simulink model "Multiplicative_Kalman_FullSystem"  (R2024a)
settings: Solver=FixedStepAuto  StartTime=0.0  StopTime=0.05  FixedStep=0.05  RelTol=1e-3
model workspace (MAT data in the model file):
  Delta_t = 0.1
  J1 = 0.1
  J2 = 0.13
  J3 = 0.05
  NoiseCov = [0.5  0  0  0  0  0; 0  0.5  0  0  0  0; 0  0  0.5  0  0  0; 0  0  0  0.5  0  0; 0  0  0  0  0.5  0; 0  0  0  0  0  0.5]
  Orbit_Incl = 51.6
  Q_identity = [0.05  0  0  0  0  0  0; 0  0.05  0  0  0  0  0; 0  0  0.05  0  0  0  0; 0  0  0  0.05  0  0  0; 0  0  0  0  0.05  0  0; 0  0  0  0  0  0.05  0; 0  0  0  0  0  0  0.05]
  Sig = Simulink.Signal
  Sig.DataType = 'auto'
  Sig.Dimensions = -1
  Sig.DimensionsMode = 'auto'
  Sig.Complexity = 'auto'
  Sig.SampleTime = -1
  Sig.SamplingMode = 'auto'
  controlRun = 1
  jd_input = 2458850
  m = 12
  n = 7
  prev_torque_input = [-64.2967060108; -71.2243432344; 28.1607266772]
  q_ff_in = [0.768047679347 -0.000607853097706 0.000738246502685 -0.640391948541]
  s_input = [0.137051174928  0.0116066773861  -0.0542772430241  -0.00220576200479  0.020662624682  0.00686951080627  -0.0162011450578; 0.0116066773861  0.107983296464  -0.0145776929418  0.0130790098983  0.00989864547201  0.00877956547813  -0.035726111281; -0.0542772430241  -0.0145776929418  0.21725961434  0.00684779520177  -0.000688284054  0.0459642589433  0.0525533115973; -0.00220576200479  0.0130790098983  0.00684779520177  0.0990005723767  0.00578790743461  -0.0243617056061  0.0483202294691; 0.020662624682  0.00989864547201  -0.000688284054  0.00578790743461  0.308218607973  0.0117877585438  0.007502538117; 0.00686951080627  0.00877956547813  0.0459642589433  -0.0243617056061  0.0117877585438  0.223868115179  0.12082283608; -0.0162011450578  -0.035726111281  0.0525533115973  0.0483202294691  0.007502538117  0.12082283608  0.257056619364]
  s_input_cons = [1.94870414  1.25588909  1.4416761  1.0780205  1.49168854  1.53894753  1.37981514; 1.25588909  2.30599344  1.57766712  1.62980068  1.46050557  1.31460547  1.13813509; 1.4416761  1.57766712  1.70958392  1.12140846  1.38322267  1.58836736  1.34392315; 1.0780205  1.62980068  1.12140846  1.77837393  1.21690337  0.94427956  1.46043147; 1.49168854  1.46050557  1.38322267  1.21690337  2.06327445  1.39185931  1.33424815; 1.53894753  1.31460547  1.58836736  0.94427956  1.39185931  2.02772691  1.7277207; 1.37981514  1.13813509  1.34392315  1.46043147  1.33424815  1.7277207  2.16380015]
  savedTorque = [38.852508509; 88.5991027354; -25.3116885458]
  t_step = 0.05
  v_icrf_input = [-2750.79999513 6666.40000211 2573.40000745]
  x_icrf_input = [3649699.96179 3308200.09259 -4676599.96426]
  x_icrf_input_cons = [3649700 3308200 -4676600]
  x_input = [-0.111705467946; -0.70150298408; -0.0584495584026; 0.701426475748; -148025.938056; -259659.807923; 192872.307113]
  x_input_cons = [0.2; 0.6; 0.5; 0.59160797831; 0.1; 0.4; 0.9]
libraries: aerolibsatdyn x1, aerolibtransform2 x1, aerolibutil x1
settings Model: Creator=alenachan  LastModifiedBy=alenachan

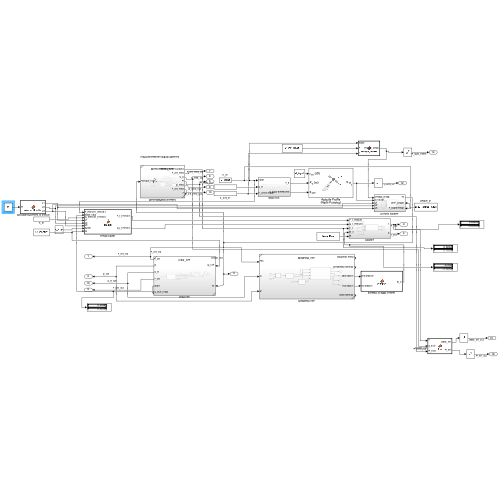
[thumbnail: Simulink's stored preview of the top-level diagram]
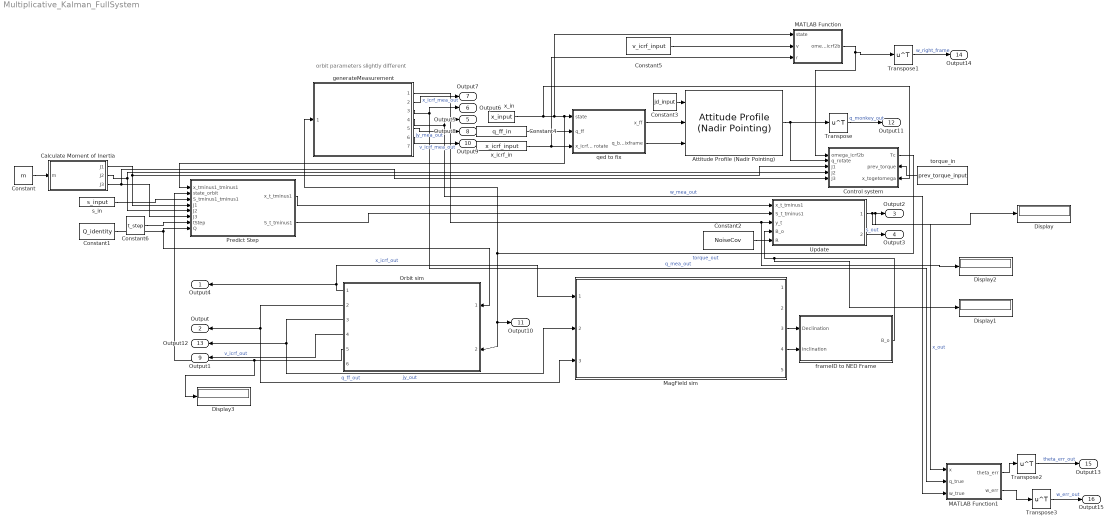
== system Multiplicative_Kalman_FullSystem ==
  note: orbit parameters slightly different
  " Calculate Moment of Inertia" : MATLAB Function  Priority=10  TreatAsAtomicUnit=on
  Attitude Profile (Nadir Pointing) : aerolibsatdyn/Attitude Profile (Nadir Pointing)  Priority=3  outputError=on  outputFinalAttitude=off  portFrame=Fixed-frame  pointingMode=Point at nadir  celestialTarget=Sun  tunablePointing=off  primaryAlignmentSrc=Dialog  primaryAlignment=[0 0 1]  secondaryAlignmentSrc=Dialog  secondaryAlignment=[1 0 0]  constraintFrame=ICRF  primaryConstraintSrc=Dialog  primaryConstraint=[1 0 0]  secondaryConstraintSrc=Dialog  secondaryConstraint=[0 1 0]
  Constant : Constant  Value=m
  Constant1 : Constant  Value=Q_identity
  Constant2 : Constant  Value=NoiseCov
  Constant3 : Constant  Value=jd_input
  Constant4 : Constant  Value=q_ff_in
  Constant5 : Constant  Value=v_icrf_input
  Constant6 : Constant  Value=t_step
  Control system : Subsystem  Priority=4
      settings: PortSchema="{\"entries\":[{\"content\":{\"sides\":[{\"content\":{\"connectorIds\":[\"In1\",\"In2\",\"In3\",\"In4\",\"In5\"]},\"type\":\"ConnectorPlacement.EquallySpacedRectSide\",\"uuid\":\"8eb5f269-cc65-4267-936a-9f0f4ccd4d18\"},{\"content\":{\"connectorIds\":[\"Out1\",\"In6\",\"In7\"],\"side\":\"RIGHT\"},\"type\":\"ConnectorPlacement.EquallySpacedRectSide\",\"uuid\":\"3df96c14-e4ae-45ba-8fc0-de3a9fdcf55a\"},{\"content\":{\"side\":\"TOP\"},\"type\":\"ConnectorPlacement.EquallySpacedRectSide\",\"uuid\":\"e3effbcc-2fcc-4dea-811c-5aa639521533\"}]},\"type\":\"ConnectorPlacement.EquallySpacedConnector\",\"uuid\":\"93bbc224-b85a-4291-8bf8-2645c40efc9b\"}],\"packageUris\":[\"http://schema.mathworks.com/mf0/Connector/R2020b\"],\"version\":\"1.0\"}"
  Display{,1..3} (4 alike) : Display
  MATLAB Function : MATLAB Function  TreatAsAtomicUnit=on
  MATLAB Function1 : MATLAB Function  TreatAsAtomicUnit=on
  MagField sim : Subsystem  Priority=8  ReferencedSubsystem=MagField_sim
  Orbit sim : Subsystem  Priority=7  ReferencedSubsystem=Orbit_sim
  Predict Step : MATLAB Function  Priority=11  TreatAsAtomicUnit=on
  Transpose{,1..3} (4 alike) : Math  Operator=transpose
  Update : Subsystem  Priority=12
  frameID to NED Frame : MATLAB Function  Priority=9  TreatAsAtomicUnit=on
  generateMeasurement : Subsystem  Priority=5  ReferencedSubsystem=Measurement_sim
  qed to fix : Subsystem  Priority=2
  s_in : Constant  Priority=1  Value=s_input
  torque_in : Constant  Value=prev_torque_input
  x_icrf_in : Constant  Value=x_icrf_input
  x_in : Constant  Value=x_input
  Output4 : Outport
  Output : Outport  Port=2
  Output2 : Outport  Port=3
  Output3 : Outport  Port=4
  Output5 : Outport  Port=5
  Output6 : Outport  Port=6
  Output7 : Outport  Port=7
  Output8 : Outport  Port=8
  Output1 : Outport  Port=9
  Output9 : Outport  Port=10
  Output10 : Outport  Port=11
  Output11 : Outport  Port=12
  Output12 : Outport  Port=13
  Output14 : Outport  Port=14
  Output13 : Outport  Port=15
  Output15 : Outport  Port=16
  wires:
  Control system/1(Tc) -> Output10/1, Orbit sim/2, generateMeasurement/1  "torque_out"
  MagField sim/3 -> frameID to NED Frame/1(Declination)
  MagField sim/4 -> frameID to NED Frame/2(Inclination)
  frameID to NED Frame/1(B_o) -> Display1/1, Update/4(B_o)
  Orbit sim/2 -> MagField sim/3, Output/1  "jy_out"
  Orbit sim/1 -> MagField sim/1, Output4/1  "x_icrf_out"
  Constant/1 -> " Calculate Moment of Inertia"/1(m)
  " Calculate Moment of Inertia"/1(J1) -> Predict Step/4(J1), Control system/3(J1)
  " Calculate Moment of Inertia"/2(J2) -> Control system/4(J2), Predict Step/5(J2)
  " Calculate Moment of Inertia"/3(J3) -> Predict Step/6(J3), Control system/5(J3)
  Constant1/1 -> Orbit sim/1, Predict Step/8(Q)
  x_in/1 -> Control system/7(x_togetomega), MATLAB Function/1(state), Predict Step/1(x_tminus1_tminus1), qed to fix/1(state)
  s_in/1 -> Predict Step/3(S_tminus1_tminus1)
  x_icrf_in/1 -> MATLAB Function/3(r), qed to fix/3(x_icrf to rotate)
  Predict Step/1(x_t_tminus1) -> Update/1(x_t_tminus1)
  Predict Step/2(S_t_tminus1) -> Update/2(S_t_tminus1)
  generateMeasurement/1 -> Display2/1, Update/3(y_t)
  Constant2/1 -> Update/5(R)
  Update/1(1) -> MATLAB Function1/1(x), Display/1, Output2/1  "x_out"
  Update/2(2) -> Output3/1  "s_out"
  Orbit sim/3 -> MagField sim/2, Output12/1  "q_ff_out"
  generateMeasurement/2 -> Output7/1  "x_icrf_mea_out"
  generateMeasurement/5 -> Output8/1  "jy_mea_out"
  Orbit sim/4 -> Output1/1  "v_icrf_out"
  generateMeasurement/6 -> Output9/1  "v_icrf_mea_out"
  torque_in/1 -> Control system/6(prev_torque)
  Transpose/1 -> Output11/1  "q_monkey_out"
  Constant3/1 -> Attitude Profile (Nadir Pointing)/1
  qed to fix/2(q_bodyToFixframe) -> Attitude Profile (Nadir Pointing)/3
  Constant4/1 -> qed to fix/2(q_ff)
  qed to fix/1(x_ff) -> Attitude Profile (Nadir Pointing)/2
  Constant6/1 -> Predict Step/7(tStep)
  Orbit sim/5 -> Display3/1, Predict Step/2(state_orbit)
  Attitude Profile (Nadir Pointing)/1 -> Transpose/1, Control system/2(q_rotate)
  Constant5/1 -> MATLAB Function/2(v)
  MATLAB Function/1(omega_icrf2b) -> Transpose1/1, Control system/1(omega_icrf2b)
  Transpose1/1 -> Output14/1  "w_right_frame"
  Transpose2/1 -> Output13/1  "theta_err_out"
  MATLAB Function1/2(w_err) -> Transpose3/1
  Transpose3/1 -> Output15/1  "w_err_out"
  generateMeasurement/4 -> Output5/1, MATLAB Function1/3(w_true)  "w_mea_out"
  generateMeasurement/3 -> Output6/1, MATLAB Function1/2(q_true)  "q_mea_out"
  MATLAB Function1/1(theta_err) -> Transpose2/1

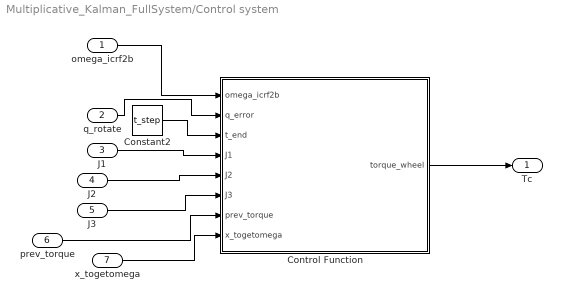
== system Multiplicative_Kalman_FullSystem/Control system ==
  omega_icrf2b : Inport
  q_rotate : Inport  Port=2
  J1 : Inport  Port=3
  J2 : Inport  Port=4
  J3 : Inport  Port=5
  prev_torque : Inport  Port=6
  x_togetomega : Inport  Port=7
  Constant2 : Constant  Value=t_step
  Control Function : MATLAB Function  TreatAsAtomicUnit=on
  Tc : Outport
  wires:
  Constant2/1 -> Control Function/3(t_end)
  Control Function/1(torque_wheel) -> Tc/1
  q_rotate/1 -> Control Function/2(q_error)
  J1/1 -> Control Function/4(J1)
  J2/1 -> Control Function/5(J2)
  J3/1 -> Control Function/6(J3)
  prev_torque/1 -> Control Function/7(prev_torque)
  x_togetomega/1 -> Control Function/8(x_togetomega)
  omega_icrf2b/1 -> Control Function/1(omega_icrf2b)

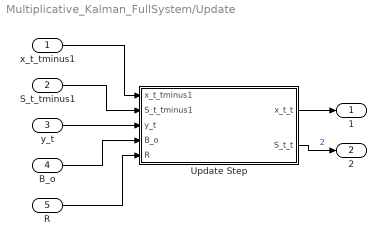
== system Multiplicative_Kalman_FullSystem/Update ==
  x_t_tminus1 : Inport
  S_t_tminus1 : Inport  Port=2
  y_t : Inport  Port=3
  B_o : Inport  Port=4
  R : Inport  Port=5
  Update Step : MATLAB Function  TreatAsAtomicUnit=on
  1 : Outport
  2 : Outport  Port=2
  wires:
  Update Step/2(S_t_t) -> 2/1  "2"
  R/1 -> Update Step/5(R)
  B_o/1 -> Update Step/4(B_o)
  Update Step/1(x_t_t) -> 1/1
  y_t/1 -> Update Step/3(y_t)
  S_t_tminus1/1 -> Update Step/2(S_t_tminus1)
  x_t_tminus1/1 -> Update Step/1(x_t_tminus1)

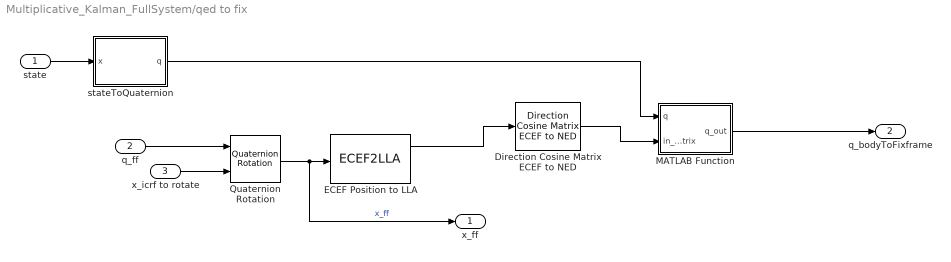
== system Multiplicative_Kalman_FullSystem/qed to fix ==
  state : Inport
  q_ff : Inport  Port=2
  x_icrf to rotate : Inport  Port=3
  Direction Cosine Matrix ECEF to NED : aerolibtransform2/Direction Cosine Matrix ECEF to NED
  ECEF Position to LLA : ECEF2LLA
  MATLAB Function : MATLAB Function  TreatAsAtomicUnit=on
  Quaternion Rotation : aerolibutil/Quaternion Rotation
  stateToQuaternion : MATLAB Function  TreatAsAtomicUnit=on
  x_ff : Outport
  q_bodyToFixframe : Outport  Port=2
  wires:
  state/1 -> stateToQuaternion/1(x)
  Quaternion Rotation/1 -> x_ff/1, ECEF Position to LLA/1  "x_ff"
  x_icrf to rotate/1 -> Quaternion Rotation/2
  ECEF Position to LLA/1 -> Direction Cosine Matrix ECEF to NED/1
  Direction Cosine Matrix ECEF to NED/1 -> MATLAB Function/2(in_matrix)
  stateToQuaternion/1(q) -> MATLAB Function/1(q)
  MATLAB Function/1(q_out) -> q_bodyToFixframe/1
  q_ff/1 -> Quaternion Rotation/1

== matlab function Multiplicative_Kalman_FullSystem/Control system/Control Function ==
  data: omega_icrf2b input; q_error input; t_end input; torque_wheel output size=[3 1]; J1 input; J2 input; J3 input; prev_torque input; x_togetomega input
function torque_wheel = fcn(omega_icrf2b, q_error, t_end, J1, J2, J3, prev_torque, x_togetomega)
coder.extrinsic("get_param");
coder.extrinsic("getVariable");
coder.extrinsic("quat2angle");
t_end = 360*t_end;

mdlWks = get_param('Multiplicative_Kalman_FullSystem','ModelWorkspace');
ctrlRn = getVariable(mdlWks,'controlRun');
if ~ctrlRn
    %disp('enter Control');

    I_sate = [J1,0,0; 0,J2,0; 0,0,J3]; % define moment of inertia (same for every wheel)
    if(norm(omega_icrf2b) > 0.5) %0.15
        disp(omega_icrf2b);
        disp('controlling rate of rotation');
        torque_wheel_calc = I_sate * (-omega_icrf2b / t_end);
        % torque_wheel_calc = -0.8*x_togetomega(5:7);
    else
        theta = abs(2*acos(q_error(1))); % magnitude
        direction = [q_error(2);q_error(3); q_error(4)]/abs(sin(theta/2)); %3d-vector
        disp('adjusting orientation');
        omega_cur_indir=dot(omega_icrf2b*t_end,direction);
        acc = ((theta - omega_cur_indir*t_end)* 2)/(t_end^2); % magnitude
        acc_directed = acc*direction; %3d-vector
        
        torque_wheel_calc = 0.9*I_sate * acc_directed + 0.1*prev_torque; % 3-d vector; 0.1 is momentum coefficient
    end

    max_torque = 100; % 0.824 * 10^(-2); %reasonable estimate from CSI document
    if norm(torque_wheel_calc) > max_torque % scale to maximum allowed magnitude
        % disp("Torque is beyond physical limit.");
        torque_wheel = (max_torque/norm(torque_wheel_calc))* torque_wheel_calc;
    else
        torque_wheel = torque_wheel_calc;
    end

    %disp(torque_wheel);

    assignin(mdlWks,'savedTorque', torque_wheel);
    assignin(mdlWks,'controlRun', true);    
else
    %disp('skipped control');
    torque_wheel = getVariable(mdlWks,'savedTorque'); % this ensures that value doesn't zero out after multiple runs
end

== matlab function Multiplicative_Kalman_FullSystem/Update/Update Step ==
  data: x_t_tminus1 input; x_t_t output; S_t_tminus1 input; y_t input; S_t_t output; B_o input; R input
function [x_t_t, S_t_t] = update(x_t_tminus1, S_t_tminus1, y_t, B_o, R)

H_out = H(x_t_tminus1, B_o);

%Kalman Gain
%temp=(H_out*S_t_tminus1*transpose(H_out) + R);
K = S_t_tminus1 * transpose(H_out)/(H_out*S_t_tminus1*transpose(H_out) + R);
%disp('update');
%Update
delta_x = K * (y_t - h_t(x_t_tminus1, B_o));
x_t_t = zeros(7,1);
x_t_t(1:4) = quatmultiply(transpose(x_t_tminus1(1:4)), transpose(delta_x(1:4)));
rest_norm = 1 - x_t_t(1)^2;
x_t_t(2:4) = x_t_t(2:4)/norm(x_t_t(2:4))*sqrt(rest_norm);
x_t_t(5:7) = x_t_tminus1(5:7)+delta_x(5:7);
% x_t_t(1:4)=x_t_t(1:4)/norm(x_t_t(1:4));
S_t_t = (eye(7) - K*H_out)*S_t_tminus1;

end

== matlab function Multiplicative_Kalman_FullSystem/Predict Step ==
  data: x_tminus1_tminus1 input; state_orbit input; x_t_tminus1 output; S_tminus1_tminus1 input; S_t_tminus1 output; J1 input; J2 input; J3 input; tStep input; Q input
function [x_t_tminus1, S_t_tminus1]= predict(x_tminus1_tminus1,state_orbit, S_tminus1_tminus1, J1,J2,J3, tStep, Q)


x_t_tminus1 = state_orbit; %use state from orbit with noise
% x_t_tminus1 = feval(f_t,x_tminus1_tminus1);
F_tminus1 = F(x_tminus1_tminus1, J1,J2,J3,tStep);
%disp('predict');
S_t_tminus1 = Q + F_tminus1 * S_tminus1_tminus1 * transpose(F_tminus1);

== matlab function Multiplicative_Kalman_FullSystem/qed to fix/MATLAB Function ==
  data: q input; in_matrix input; q_out output
function q_out= fcn(q, in_matrix)
inv_m = inv(in_matrix);
q_second = rotm2quat(inv_m);
q_first = quatconj(q);
q_out = transpose(quatmultiply(q_second,q_first));

== matlab function Multiplicative_Kalman_FullSystem/qed to fix/stateToQuaternion ==
  data: x input; q output
function q = getq(x)
q_temp = x(1:4);
q = transpose(q_temp);
end

== matlab function Multiplicative_Kalman_FullSystem/frameID to NED Frame ==
  data: Declination input; Inclination input; B_o output
function B_o= ID2NED(Declination,Inclination)

[Down_dir,Omega_dir,Other_dir] = MagID2NED(Inclination,Declination);
B_o = [Down_dir;Omega_dir;Other_dir]/norm([Down_dir,Omega_dir,Other_dir]);
%disp('enter NED')

end

== matlab function Multiplicative_Kalman_FullSystem/MATLAB Function ==
  data: state input; v input; omega_icrf2b output; r input
function omega_icrf2b = omega_frame(state,v,r)
omega_ned2b = state(5:7);
omega_icrf2ned = -cross(r,v)/norm(r)^2;
omega_icrf2b = omega_ned2b + omega_icrf2ned;

== matlab function Multiplicative_Kalman_FullSystem/MATLAB Function1 ==
  data: x input; theta_err output; q_true input; w_true input; w_err output
function [theta_err, w_err]= fcn(x, q_true, w_true)
theta_est = 2*acos(x(1));
theta_true = 2*acos(q_true(1));
theta_err = theta_est - theta_true;
w_err = transpose(x(5:7))-w_true;

== matlab function Multiplicative_Kalman_FullSystem/ Calculate Moment of Inertia ==
  data: m input; J1 output; J2 output; J3 output
function [J1,J2,J3]=momentInertia(m)
J1 = m/120;
J2 = 13*m/1200;
J3 = 5*m/1200;
coder.extrinsic("get_param");
mdlWks = get_param('Multiplicative_Kalman_FullSystem','ModelWorkspace');
assignin(mdlWks,"J1",J1)
assignin(mdlWks,"J2",J2)
assignin(mdlWks,"J3",J3)
end
